simulink model "Model_6DOF_B3_2019a"  (R2019a)
settings: Solver=FixedStepAuto  StartTime=0.0  StopTime=200  FixedStep=0.05  RelTol=1e-3
values from neighbouring files (symbols this model uses):
  Ba_0 = [0 0 0 0 0 0]    [ctrl_mode_param.m]
  Bb = 4418825.3321    [load_data.m]
  Bv_0 = [tgt_speed 0 0 0 0 0]    [ctrl_mode_param.m]
  Bx_0 = [0 0 tgt_depth 0 0 0]    [ctrl_mode_param.m]
  check_angle = 10    [ctrl_mode_param.m]
  dX_imposed = 10    [ctrl_mode_param.m]
  Ixx = 5.23e7    (= 52300000)    [load_data.m]
  Ixy = 0    [load_data.m]
  Ixz = 0    [load_data.m]
  Iyy = 1.375e9    (= 1375000000)    [load_data.m]
  Iyz = 0    [load_data.m]
  Izz = 1.367e9    (= 1367000000)    [load_data.m]
  Mb = 4418825.3321    [load_data.m]
  Seastate = 5    [ctrl_mode_param.m]    (also in run.m = 0)
  Xb = 0    [load_data.m]
  Xg = 0    [load_data.m]
  Yb = 0    [load_data.m]
  Yg = 0    [load_data.m]
  Zb = 0.4406    [load_data.m]
  Zg = 0    [load_data.m]
undefined symbols (not defined in the file or in its folder): dA_BP1, dA_BP2, dA_Hull, dA_PH, dA_Sail, dA_SProot, dA_X1a, dA_X1b, dA_X2a, dA_X2b, dA_X3a, dA_X3b, dA_X4a, dA_X4b, DoF_switch, fwrite, its, LCG_switch, m_switch, mass_switch, n_BP1, n_BP2, n_Hull, n_imposed, n_PH, n_Sail, n_SProot, n_switch, n_X1a, n_X1b, n_X2a, n_X2b, n_X3a, n_X3b, n_X4a, n_X4b, nt_BP1, nt_BP2, nt_Hull, nt_PH, nt_Sail, nt_SProot, nt_X1a, nt_X1b, nt_X2a, nt_X2b, nt_X3a, nt_X3b, nt_X4a, nt_X4b, sail_switch, target_pitch, target_y, target_yaw, target_z, Usp, vt1_BP1, vt1_BP2, vt1_Hull, vt1_PH ... (+38)
libraries: simulink x5
(part 2 of 6)

== system Model_6DOF_B3_2019a/HDM/HDM B3/Wave, Virtual Mass and Hydrostatic ==
  Bx_earth : Inport
  Bv_ship : Inport  Port=2
  SeaState : Inport  Port=3
  dLCG : Inport  Port=4
  Ba_ship : Inport  Port=5
  dX_CTRL : Inport  Port=6
  fwrite : Inport  Port=7
  Add : Sum  Inputs=+-
  CG : Constant  Value=[32.3114 0 0]
  CGi : Constant  Value=|
      | [5.0784E+00	0.0000E+00	8.0728E-03;
      | 1.1013E+01	0.0000E+00	2.5384E-01;
      | 1.7302E+01	0.0000E+00	3.0728E-01;
      | 2.5741E+01	0.0000E+00	4.1417E-01;
      | 3.4688E+01	0.0000E+00	4.1585E-01;
      | 4.2324E+01	0.0000E+00	3.2444E-01;
      | 4.9992E+01	0.0000E+00	3.3454E-01;
      | 5.7427E+01	0.0000E+00	1.7420E-02;
      | 6.3078E+01	0.0000E+00	1.8824E-02;
      | 6.6703E+01	0.0000E+00	1.1340E-02;
      | 2.5141E+01	0.0000E+00	8.6491E+00;
      | 2.1732E+01	0.0000E+00	9.7273E+00;
      | 6.3166E+01	0.0000E+00	-4.0823E-17;
      | 2.2043E+01	0.0000E+00	9.7261E+00;
      | 6.3451E+01	0.0000E+00	-6.2238E-17;
      | ]
  Cvm*dm : Constant  Value=|
      | [8.4658E+04	1.7229E+05	1.6487E+05
      | 2.3551E+04	4.3394E+05	3.6176E+05
      | 1.1585E+03	5.9767E+05	4.2996E+05
      | 1.4123E+02	1.1354E+06	6.5606E+05
      | 9.1503E+01	6.9712E+05	5.1688E+05
      | 9.6110E+01	6.7201E+05	5.1905E+05
      | 1.2163E+04	5.7818E+05	4.7547E+05
      | 3.7219E+04	3.4697E+05	3.3508E+05
      | 1.9318E+04	7.7284E+04	7.6560E+04
      | 1.5368E+04	2.6375E+04	2.6268E+04
      | 1.8312E+04	4.5870E+05	5.1108E+04
      | 3.1859E+02	1.2645E+04	3.4886E+02
      | 3.0285E+03	4.4945E+04	4.4489E+04
      | 7.9160E+02	8.8963E+02	1.3306E+04
      | 1.2115E+03	3.9547E+04	3.9205E+04
      | ]
  Demux : Demux  Outputs=3
  Demux1 : Demux  Outputs=3
  Derivative : Derivative
  Derivative1 : Derivative
  Gain : Gain
  MATLAB Function : MATLAB Function  TreatAsAtomicUnit=on
  MATLAB Function1 : MATLAB Function  TreatAsAtomicUnit=on
  Manual Switch : ManualSwitch
  Wave Particle Motions : Subsystem
  Xvm : Outport
  Yvm : Outport  Port=2
  Zvm : Outport  Port=3
  Kvm : Outport  Port=4
  Mvm : Outport  Port=5
  Nvm : Outport  Port=6
  z_eff : Outport  Port=7
  uwsXi : Outport  Port=8
  uwsCG : Outport  Port=9
  B_FM : Outport  Port=10
  wires:
  Wave Particle Motions/2(zeff) -> z_eff/1
  Bx_earth/1 -> Wave Particle Motions/2(X_earth)
  CGi/1 -> Wave Particle Motions/3(CGi)
  CG/1 -> Wave Particle Motions/4(CG)
  Wave Particle Motions/1(Rs) -> MATLAB Function/3(Rs)
  SeaState/1 -> Wave Particle Motions/5(SeaState)
  dLCG/1 -> Wave Particle Motions/6(dLCG)
  Bv_ship/1 -> Wave Particle Motions/1(U_ship)
  MATLAB Function/7(Fvm) -> Manual Switch/1  "Fvm"
  MATLAB Function/8(Mvm) -> Demux1/1  "Mvm"
  Demux/1 -> Xvm/1
  Demux/2 -> Yvm/1
  Demux/3 -> Zvm/1
  Demux1/2 -> Mvm/1
  Demux1/1 -> Kvm/1
  Demux1/3 -> Nvm/1
  Wave Particle Motions/3(uwXis) -> uwsXi/1
  Wave Particle Motions/4(uwsCG) -> uwsCG/1, Derivative/1
  Cvm*dm/1 -> Gain/1
  Derivative/1 -> MATLAB Function1/1(awsCG)
  Ba_ship/1 -> MATLAB Function1/2(asCG)
  Manual Switch/1 -> Demux/1
  MATLAB Function1/1(Fvm) -> Manual Switch/2
  Wave Particle Motions/5(uws) -> Add/1
  Wave Particle Motions/6(urs) -> Add/2
  Add/1 -> Derivative1/1
  Derivative1/1 -> MATLAB Function/2(Awrs)  "d/dt(aw-ar)"
  Wave Particle Motions/7(B_FM) -> B_FM/1
  Gain/1 -> MATLAB Function/1(cvm)
  dX_CTRL/1 -> Wave Particle Motions/7(dX_CTRL)
  fwrite/1 -> Wave Particle Motions/8(fwrite)

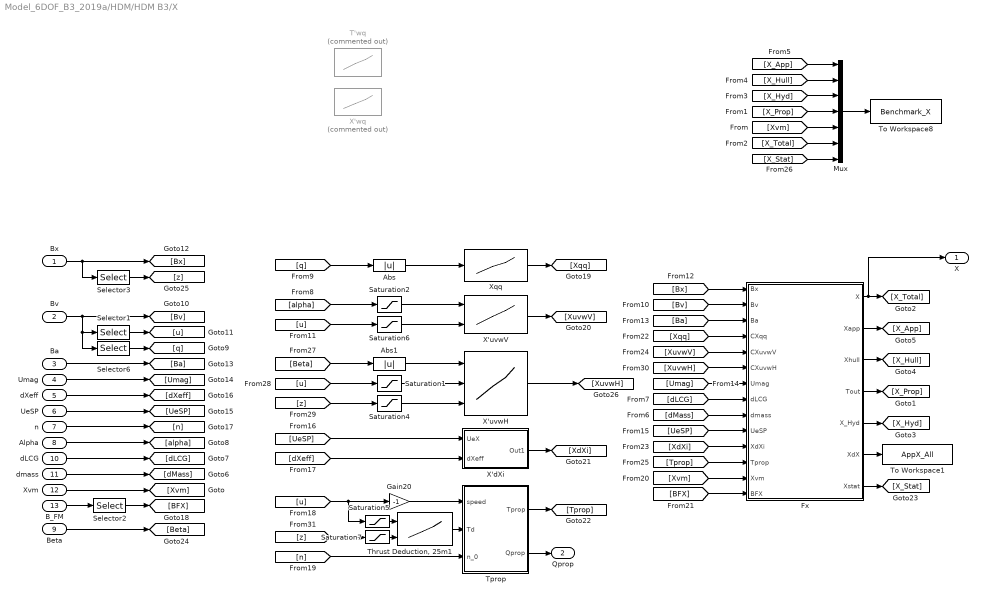
== system Model_6DOF_B3_2019a/HDM/HDM B3/X ==
  Bx : Inport
  Bv : Inport  Port=2
  Ba : Inport  Port=3
  Umag : Inport  Port=4
  dXeff : Inport  Port=5
  UeSP : Inport  Port=6
  n : Inport  Port=7
  Alpha : Inport  Port=8
  Beta : Inport  Port=9
  dLCG : Inport  Port=10
  dmass : Inport  Port=11
  Xvm : Inport  Port=12
  B_FM : Inport  Port=13
  Abs : Abs
  Abs1 : Abs
  Fx : MATLAB Function  TreatAsAtomicUnit=on
  Gain20 : Gain  Gain=-1
  Mux : Mux  Inputs=7
  Saturation1 : Saturate  UpperLimit=-1.543332  LowerLimit=-5.14444
  Saturation2 : Saturate  UpperLimit=30  LowerLimit=-30
  Saturation4 : Saturate  UpperLimit=-13.8724  LowerLimit=-35.0624
  Saturation5 : Saturate  UpperLimit=-13.8724  LowerLimit=-36.3724
  Saturation6 : Saturate  UpperLimit=-1.543332  LowerLimit=-5.14444
  Saturation7 : Saturate  UpperLimit=-1.54333333  LowerLimit=-5.14444
  Selector1 : Selector  InputPortWidth=6  IndexOptions=Index vector (dialog)  Indices=1  OutputSizes=1
  Selector2 : Selector  InputPortWidth=6  IndexOptions=Index vector (dialog)  Indices=1  OutputSizes=1
  Selector3 : Selector  InputPortWidth=6  IndexOptions=Index vector (dialog)  Indices=3  OutputSizes=1
  Selector6 : Selector  InputPortWidth=6  IndexOptions=Index vector (dialog)  Indices=5  OutputSizes=1
  T'wq : Lookup_n-D  Commented=on  BreakpointsForDimension1=|  BreakpointsForDimension2=|  Table=|  InternalRulePriority=Speed  RndMeth=Simplest  InputSameDT=on
      BreakpointsForDimension1=|
      | [-2.5000E-02
      | -2.0000E-02
      | -1.5000E-02
      | -1.0000E-02
      | -5.0000E-03
      | 0.0000E+00
      | 5.0000E-03
      | ]
      BreakpointsForDimension2=|
      | [-7.71666
      | -5.14444
      | -3.086664]
      Table=|
      | reshape([-2.7354E-04
      | -2.2597E-04
      | -1.7840E-04
      | -1.3083E-04
      | -8.3252E-05
      | -3.5680E-05
      | 1.1893E-05
      | -9.4081E-05
      | -7.5784E-05
      | -5.7487E-05
      | -3.9189E-05
      | -2.0892E-05
      | -2.5949E-06
      | 1.5702E-05
      | -1.4962E-04
      | -1.2035E-04
      | -9.1070E-05
      | -6.1795E-05
      | -3.2519E-05
      | -3.2436E-06
      | 2.6032E-05
      | ],[7,3])
  "Thrust Deduction, 25m1" : Lookup_n-D  BreakpointsForDimension1=|  BreakpointsForDimension2=[-5.14444 -3.086664 -1.543332]  Table=|  InternalRulePriority=Speed  RndMeth=Simplest  InputSameDT=on
      BreakpointsForDimension1=|
      | [-36.3724
      | -18.3724
      | -15.3724
      | -13.8724]
      Table=|
      | reshape([0.245958
      | 0.251311246
      | 0.25251
      | 0.251322
      | 0.2444134
      | 0.2498597
      | 0.2509219
      | 0.2498992
      | 0.2496
      | 0.2594532
      | 0.257802
      | 0.2475762],[4,3])
  To Workspace1 : ToWorkspace  VariableName=AppX_All  SaveFormat=Timeseries  SampleTime=-1
  To Workspace8 : ToWorkspace  VariableName=Benchmark_X  SaveFormat=Timeseries  SampleTime=-1
  Tprop : MATLAB Function  TreatAsAtomicUnit=on
  X'dXi : Subsystem
  X'uvwH : Lookup_n-D  NumberOfTableDimensions=3  BreakpointsForDimension1=|  BreakpointsForDimension2=|  BreakpointsForDimension3=|  Table=|  InternalRulePriority=Speed  RndMeth=Simplest  InputSameDT=on
      BreakpointsForDimension1=|
      | [0
      | 4
      | 8
      | 12]
      BreakpointsForDimension2=|
      | [-5.1444
      | -3.08664
      | -1.54332]
      Table=|
      | reshape([0.0000000E+00
      | 8.7490400E-05
      | -4.2970032E-04
      | -8.6882993E-04
      | 0.0000000E+00
      | 9.2255510E-05
      | -3.6462757E-04
      | -8.6516720E-04
      | 0.0000000E+00
      | -8.0508235E-05
      | -3.3610820E-04
      | -9.1603355E-04
      | 0.0000000E+00
      | -9.0915847E-05
      | -3.9252667E-04
      | -9.2068441E-04
      | 0.0000000E+00
      | -1.0407599E-04
      | -3.8836462E-04
      | -9.1865822E-04
      | 0.0000000E+00
      | -8.4723950E-05
      | -3.5324770E-04
      | -9.7126434E-04
      | 0.0000000E+00
      | -9.3766627E-05
      | -4.1342843E-04
      | -9.4161914E-04
      | 0.0000000E+00
      | -1.0916277E-04
      | -4.0683220E-04
      | -9.6707684E-04
      | 0.0000000E+00
      | -8.8664811E-05
      | -3.7605406E-04
      | -9.4194453E-04
      | 0.0000000E+00
      | -9.2876985E-05
      | -4.0365964E-04
      | -9.3239814E-04
      | 0.0000000E+00
      | -1.1414747E-04
      | -4.4323139E-04
      | -1.0049645E-03
      | 0.0000000E+00
      | -9.4615234E-05
      | -4.9251136E-04
      | -9.8471513E-04],[4,3,4])
      BreakpointsForDimension3=|
      | [-35.0624 -18.3724 -15.3724 -13.8724
      | ]
  X'uvwV : Lookup_n-D  BreakpointsForDimension1=|  BreakpointsForDimension2=|  Table=|  InternalRulePriority=Speed  RndMeth=Simplest  InputSameDT=on
      BreakpointsForDimension1=|
      | [-12
      | -8
      | -4
      | 0
      | 4
      | 8
      | 12]
      BreakpointsForDimension2=|
      | [-5.1444
      | -3.08664
      | -1.54332]
      Table=|
      | reshape([8.5556500E-04
      | 9.0045500E-04
      | 9.7379500E-04
      | 1.0292250E-03
      | 1.0286950E-03
      | 9.7963500E-04
      | 1.0147450E-03
      | 9.0637500E-04
      | 9.3710500E-04
      | 1.0133950E-03
      | 1.0723650E-03
      | 1.0693650E-03
      | 1.0284650E-03
      | 1.1084650E-03
      | 9.8653120E-04
      | 9.9350120E-04
      | 1.0534412E-03
      | 1.1098412E-03
      | 1.1115412E-03
      | 1.0836412E-03
      | 1.1582412E-03],[7,3])
  X'wq : Lookup_n-D  Commented=on  BreakpointsForDimension1=|  BreakpointsForDimension2=[-7.71666 -5.14444 -3.086664 -1.543332]  Table=|  InternalRulePriority=Speed  RndMeth=Simplest  InputSameDT=on
      BreakpointsForDimension1=|
      | [-2.5000E-02
      | -2.0000E-02
      | -1.5000E-02
      | -1.0000E-02
      | -5.0000E-03
      | 0.0000E+00
      | 5.0000E-03
      | ]
      Table=|
      | reshape([2.0716E-04
      | 1.9060E-04
      | 1.7404E-04
      | 1.5748E-04
      | 1.4091E-04
      | 1.2435E-04
      | 1.0779E-04
      | 1.3610E-04
      | 1.1954E-04
      | 1.0298E-04
      | 8.6416E-05
      | 6.9855E-05
      | 5.3295E-05
      | 3.6734E-05
      | 1.5577E-04
      | 1.2817E-04
      | 1.0057E-04
      | 7.2967E-05
      | 4.5366E-05
      | 1.7765E-05
      | -9.8361E-06
      | 1.4245E-04
      | 1.1485E-04
      | 8.7244E-05
      | 5.9643E-05
      | 3.2042E-05
      | 4.4412E-06
      | -2.3160E-05
      | ],[7,4])
  Xqq : Lookup_n-D  NumberOfTableDimensions=1  BreakpointsForDimension1=|  Table=|  InternalRulePriority=Speed  RndMeth=Simplest  InputSameDT=on
      BreakpointsForDimension1=|
      | [-0.02
      | -0.015
      | -0.012958963
      | -0.009719222
      | -0.006479482
      | -0.003239741
      | -0.00161987
      | -0.000647948
      | 0.000647948
      | 0.00161987
      | 0.003239741
      | 0.006479482
      | 0.009719222
      | 0.012958963
      | 0.015
      | 0.02
      | ]
      Table=|
      | [1.5581E-04
      | 1.1369E-04
      | 2.0348E-04
      | 4.5268E-04
      | 3.8456E-04
      | 9.9241E-05
      | 3.8998E-04
      | 9.1300E-05
      | -3.1574E-04
      | -7.9139E-05
      | -9.0517E-04
      | -4.4764E-04
      | -5.9612E-04
      | -5.5873E-04
      | -5.9343E-04
      | -5.5869E-04
      | ]
  X : Outport
  Qprop : Outport  Port=2
  wires:
  Saturation2/1 -> X'uvwV/1
  Gain20/1 -> Tprop/1(speed)
  Fx/1(X) -> [X_Total], X/1
  [u] -> Saturation5/1, Gain20/1
  [q] -> Abs/1
  Abs/1 -> Xqq/1
  "Thrust Deduction, 25m1"/1 -> Tprop/2(Td)
  Saturation6/1 -> X'uvwV/2
  Mux/1 -> To Workspace8/1
  Fx/6(XdX) -> To Workspace1/1
  B_FM/1 -> Selector2/1
  Fx/7(Xstat) -> [X_Stat]
  [Xvm] -> Mux/5
  Fx/4(Tout) -> [X_Prop]
  [X_Prop] -> Mux/4
  [X_Total] -> Mux/6
  [X_Hyd] -> Mux/3
  Fx/5(X_Hyd) -> [X_Hyd]
  [X_Hull] -> Mux/2
  Fx/3(Xhull) -> [X_Hull]
  Fx/2(Xapp) -> [X_App]
  [X_App] -> Mux/1
  [dMass] -> Fx/9(dmass)
  dmass/1 -> [dMass]
  [dLCG] -> Fx/8(dLCG)
  dLCG/1 -> [dLCG]
  [alpha] -> Saturation2/1
  Alpha/1 -> [alpha]
  Bv/1 -> [Bv], Selector6/1, Selector1/1
  Selector6/1 -> [q]
  [Bv] -> Fx/2(Bv)
  [u] -> Saturation6/1
  Selector1/1 -> [u]
  [Bx] -> Fx/1(Bx)
  Bx/1 -> [Bx], Selector3/1
  [Ba] -> Fx/3(Ba)
  Ba/1 -> [Ba]
  [Umag] -> Fx/7(Umag)
  Umag/1 -> [Umag]
  [UeSP] -> Fx/10(UeSP)
  UeSP/1 -> [UeSP]
  [UeSP] -> X'dXi/1(UeX)
  [dXeff] -> X'dXi/2(dXeff)
  dXeff/1 -> [dXeff]
  n/1 -> [n]
  [n] -> Tprop/3(n_0)
  Xvm/1 -> [Xvm]
  [Xvm] -> Fx/13(Xvm)
  Selector2/1 -> [BFX]
  [BFX] -> Fx/14(BFX)
  [Xqq] -> Fx/4(CXqq)
  Xqq/1 -> [Xqq]
  X'uvwV/1 -> [XuvwV]
  X'dXi/1(Out1) -> [XdXi]
  [XdXi] -> Fx/11(XdXi)
  [XuvwV] -> Fx/5(CXuvwV)
  Tprop/1(Tprop) -> [Tprop]
  [Tprop] -> Fx/12(Tprop)
  [X_Stat] -> Mux/7
  Beta/1 -> [Beta]
  Abs1/1 -> X'uvwH/1
  [Beta] -> Abs1/1
  [u] -> Saturation1/1
  Saturation1/1 -> X'uvwH/2
  Selector3/1 -> [z]
  [z] -> Saturation4/1
  Saturation4/1 -> X'uvwH/3
  X'uvwH/1 -> [XuvwH]
  [XuvwH] -> Fx/6(CXuvwH)
  Saturation5/1 -> "Thrust Deduction, 25m1"/1
  Saturation7/1 -> "Thrust Deduction, 25m1"/2
  [z] -> Saturation7/1
  Tprop/2(Qprop) -> Qprop/1

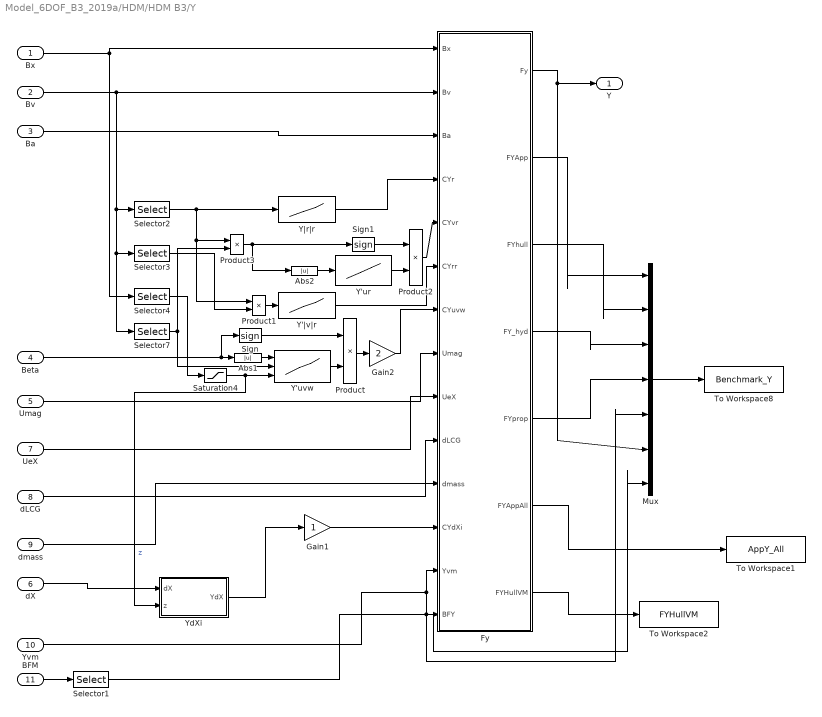
== system Model_6DOF_B3_2019a/HDM/HDM B3/Y ==
  Bx : Inport
  Bv : Inport  Port=2
  Ba : Inport  Port=3
  Beta : Inport  Port=4
  Umag : Inport  Port=5
  dX : Inport  Port=6
  UeX : Inport  Port=7
  dLCG : Inport  Port=8
  dmass : Inport  Port=9
  Yvm : Inport  Port=10
  BFM : Inport  Port=11
  Abs1 : Abs
  Abs2 : Abs
  Fy : MATLAB Function  TreatAsAtomicUnit=on
  Gain1 : Gain
  Gain2 : Gain  Gain=2
  Mux : Mux  Inputs=7
  Product{,1..3} (4 alike) : Product
  Saturation4 : Saturate  UpperLimit=-13.8724  LowerLimit=-35.0624
  Selector1 : Selector  InputPortWidth=6  IndexOptions=Index vector (dialog)  Indices=2  OutputSizes=1
  Selector2 : Selector  InputPortWidth=6  IndexOptions=Index vector (dialog)  Indices=6  OutputSizes=1
  Selector3 : Selector  InputPortWidth=6  IndexOptions=Index vector (dialog)  Indices=2  OutputSizes=1
  Selector4 : Selector  InputPortWidth=6  IndexOptions=Index vector (dialog)  Indices=3  OutputSizes=1
  Selector7 : Selector  InputPortWidth=6  IndexOptions=Index vector (dialog)  Indices=1  OutputSizes=1
  Sign : Signum
  Sign1 : Signum
  To Workspace1 : ToWorkspace  VariableName=AppY_All  SaveFormat=Timeseries  SampleTime=-1
  To Workspace2 : ToWorkspace  VariableName=FYHullVM  SaveFormat=Timeseries  SampleTime=-1
  To Workspace8 : ToWorkspace  VariableName=Benchmark_Y  SaveFormat=Timeseries  SampleTime=-1
  Y'ur : Lookup_n-D  NumberOfTableDimensions=1  BreakpointsForDimension1=|  Table=|  InternalRulePriority=Speed  RndMeth=Simplest  InputSameDT=on
      BreakpointsForDimension1=|
      | [0.03999989
      | 0.079999993
      | 0.11999963
      | 0.15999956]
      Table=|
      | [-5.2094E-04
      | -1.0594E-03
      | -1.5649E-03
      | -2.0981E-03]
  Y'uvw : Lookup_n-D  NumberOfTableDimensions=3  BreakpointsForDimension1=|  BreakpointsForDimension2=|  BreakpointsForDimension3=|  Table=|  InternalRulePriority=Speed  RndMeth=Simplest  InputSameDT=on
      BreakpointsForDimension1=|
      | [0
      | 4
      | 8
      | 12]
      BreakpointsForDimension2=|
      | [-5.1444E+00
      | -3.0866E+00
      | -1.5433E+00
      | ]
      Table=|
      | reshape([0.0000000E+00
      | -5.0280621E-03
      | -9.4175348E-03
      | -1.4397458E-02
      | 0.0000000E+00
      | -5.0037454E-03
      | -9.1645405E-03
      | -1.4507402E-02
      | 0.0000000E+00
      | -4.2819107E-03
      | -9.0361786E-03
      | -1.4507235E-02
      | 0.0000000E+00
      | -4.7723270E-03
      | -9.7378407E-03
      | -1.5377541E-02
      | 0.0000000E+00
      | -4.7276301E-03
      | -9.6949815E-03
      | -1.5393721E-02
      | 0.0000000E+00
      | -4.5359209E-03
      | -9.4966039E-03
      | -1.6947859E-02
      | 0.0000000E+00
      | -5.1295007E-03
      | -1.0575377E-02
      | -1.6672924E-02
      | 0.0000000E+00
      | -4.9811404E-03
      | -1.0209461E-02
      | -1.6298327E-02
      | 0.0000000E+00
      | -4.7780219E-03
      | -1.0008968E-02
      | -1.6115181E-02
      | 0.0000000E+00
      | -5.7252015E-03
      | -1.1973447E-02
      | -1.9152812E-02
      | 0.0000000E+00
      | -5.2128737E-03
      | -1.0845978E-02
      | -1.7281669E-02
      | 0.0000000E+00
      | -4.9979037E-03
      | -1.0845685E-02
      | -1.6944141E-02],[4,3,4])
      BreakpointsForDimension3=|
      | [-35.0624 -18.3724 -15.3724 -13.8724
      | ]
  Y'|v|r : Lookup_n-D  NumberOfTableDimensions=1  BreakpointsForDimension1=|  Table=|  InternalRulePriority=Speed  RndMeth=Simplest  InputSameDT=on
      BreakpointsForDimension1=|
      | [-0.0015
      | -0.0012
      | -0.0009
      | -0.0006
      | -0.0003
      | -0.0001
      | 0.0001
      | 0.0003
      | 0.0006
      | 0.0009
      | 0.0012
      | 0.0015]
      Table=|
      | [-2.9784E-01
      | -2.6725E-01
      | -2.3292E-01
      | -2.0077E-01
      | -1.1489E-01
      | -7.6673E-03
      | -7.5516E-03
      | -1.1617E-01
      | -2.0077E-01
      | -2.9128E-01
      | -3.5974E-01
      | -4.7839E-01]
  YdXi : Subsystem
  Y|r|r : Lookup_n-D  NumberOfTableDimensions=1  BreakpointsForDimension1=|  Table=|  InternalRulePriority=Speed  RndMeth=Simplest  InputSameDT=on
      BreakpointsForDimension1=|
      | [-0.02
      | -0.015
      | -0.012958963
      | -0.009719222
      | -0.006479482
      | -0.003239741
      | -0.00161987
      | -0.000647948
      | 0.000647948
      | 0.00161987
      | 0.003239741
      | 0.006479482
      | 0.009719222
      | 0.012958963
      | 0.015
      | 0.02
      | ]
      Table=|
      | [3.6478E-03
      | 3.8686E-03
      | 3.4313E-03
      | 4.0790E-03
      | 3.9500E-03
      | 3.6018E-03
      | 3.6796E-03
      | 3.5502E-03
      | 3.4310E-03
      | 3.4872E-03
      | 4.2239E-03
      | 4.0934E-03
      | 3.0314E-03
      | 2.5726E-03
      | 2.9188E-03
      | 2.7740E-03
      | ]
  Y : Outport
  wires:
  Selector7/1 -> Product3/2, Y'uvw/2
  Beta/1 -> Sign/1, Abs1/1
  Bv/1 -> Selector7/1, Selector3/1, Selector2/1, Fy/2(Bv)
  Umag/1 -> Fy/8(Umag)
  Bx/1 -> Selector4/1, Fy/1(Bx)
  UeX/1 -> Fy/9(UeX)
  Selector3/1 -> Product1/2
  Ba/1 -> Fy/3(Ba)
  dLCG/1 -> Fy/10(dLCG)
  dmass/1 -> Fy/11(dmass)
  dX/1 -> YdXi/1(dX)
  Product3/1 -> Abs2/1, Sign1/1
  Product1/1 -> Y'|v|r/1
  Selector2/1 -> Product1/1, Product3/1, Y|r|r/1
  Y'|v|r/1 -> Fy/6(CYrr)
  Fy/1(Fy) -> Mux/6, Y/1
  Y|r|r/1 -> Fy/4(CYr)
  Y'ur/1 -> Product2/2
  Selector4/1 -> Saturation4/1
  Y'uvw/1 -> Product/2
  Sign/1 -> Product/1
  Abs1/1 -> Y'uvw/1
  Product2/1 -> Fy/5(CYvr)
  Sign1/1 -> Product2/1
  Abs2/1 -> Y'ur/1
  YdXi/1(YdX) -> Gain1/1
  Product/1 -> Gain2/1
  Gain2/1 -> Fy/7(CYuvw)
  Yvm/1 -> Mux/5, Fy/13(Yvm)
  Mux/1 -> To Workspace8/1
  Fy/2(FYApp) -> Mux/1
  Fy/3(FYhull) -> Mux/2
  Fy/4(FY_hyd) -> Mux/3
  Fy/5(FYprop) -> Mux/4
  Fy/6(FYAppAll) -> To Workspace1/1
  BFM/1 -> Selector1/1
  Selector1/1 -> Mux/7, Fy/14(BFY)
  Fy/7(FYHullVM) -> To Workspace2/1
  Saturation4/1 -> Y'uvw/3, YdXi/2(z)  "z"
  Gain1/1 -> Fy/12(CYdXi)

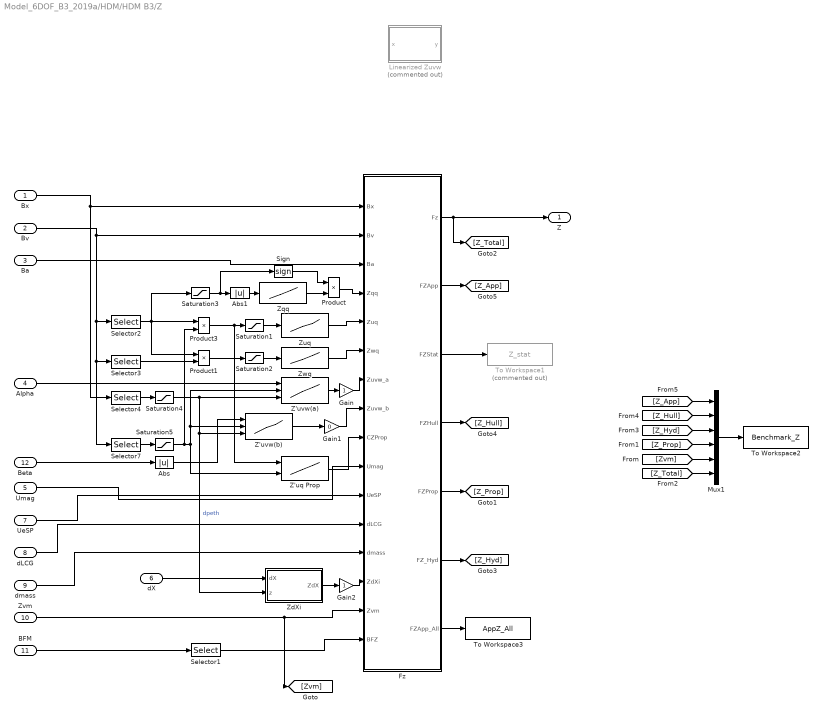
== system Model_6DOF_B3_2019a/HDM/HDM B3/Z ==
  Bx : Inport
  Bv : Inport  Port=2
  Ba : Inport  Port=3
  Alpha : Inport  Port=4
  Umag : Inport  Port=5
  dX : Inport  Port=6
  UeSP : Inport  Port=7
  dLCG : Inport  Port=8
  dmass : Inport  Port=9
  Zvm : Inport  Port=10
  BFM : Inport  Port=11
  Beta : Inport  Port=12
  Abs : Abs
  Abs1 : Abs
  Fz : MATLAB Function  TreatAsAtomicUnit=on
  Gain : Gain
  Gain1 : Gain  Gain=0
  Gain2 : Gain
  Linearized Zuvw : MATLAB Function  Commented=on  TreatAsAtomicUnit=on
  Mux1 : Mux  Inputs=6
  Product : Product
  Product1 : Product
  Product3 : Product
  Saturation1 : Saturate  UpperLimit=0.04  LowerLimit=-0.04
  Saturation2 : Saturate  UpperLimit=0.0015  LowerLimit=-0.0015
  Saturation3 : Saturate  UpperLimit=0.02  LowerLimit=-0.02
  Saturation4 : Saturate  UpperLimit=-13.8724  LowerLimit=-35.0624
  Saturation5 : Saturate  UpperLimit=-1.5433E+00  LowerLimit=-5.14444
  Selector1 : Selector  InputPortWidth=6  IndexOptions=Index vector (dialog)  Indices=3  OutputSizes=1
  Selector2 : Selector  InputPortWidth=6  IndexOptions=Index vector (dialog)  Indices=5  OutputSizes=1
  Selector3 : Selector  InputPortWidth=6  IndexOptions=Index vector (dialog)  Indices=3  OutputSizes=1
  Selector4 : Selector  InputPortWidth=6  IndexOptions=Index vector (dialog)  Indices=3  OutputSizes=1
  Selector7 : Selector  InputPortWidth=6  IndexOptions=Index vector (dialog)  Indices=1  OutputSizes=1
  Sign : Signum
  To Workspace1 : ToWorkspace  Commented=on  VariableName=Z_stat  SaveFormat=Timeseries  SampleTime=-1
  To Workspace2 : ToWorkspace  VariableName=Benchmark_Z  SaveFormat=Timeseries  SampleTime=-1
  To Workspace3 : ToWorkspace  VariableName=AppZ_All  SaveFormat=Timeseries  SampleTime=-1
  Z'uq Prop : Lookup_n-D  BreakpointsForDimension1=|  BreakpointsForDimension2=[-7.71666 -5.14444 -3.086664 -1.543332]  Table=|  InternalRulePriority=Speed  RndMeth=Simplest  InputSameDT=on
      BreakpointsForDimension1=|
      | [-2.0E-01
      | -1.5E-01
      | -1.0E-01
      | -5.0E-02
      | 0.0E+00
      | 5.0E-02
      | 1.0E-01
      | 1.5E-01
      | 2.0E-01
      | ]
      Table=|
      | reshape([1.3913E-04
      | 1.0452E-04
      | 6.9900E-05
      | 3.5283E-05
      | 6.6700E-07
      | -3.3949E-05
      | -6.8566E-05
      | -1.0318E-04
      | -1.3780E-04
      | 2.8914E-04
      | 2.1702E-04
      | 1.4490E-04
      | 7.2785E-05
      | 6.6700E-07
      | -7.1451E-05
      | -1.4357E-04
      | -2.1569E-04
      | -2.8780E-04
      | 1.1606E-04
      | 8.7208E-05
      | 5.8361E-05
      | 2.9514E-05
      | 6.6700E-07
      | -2.8180E-05
      | -5.7027E-05
      | -8.5874E-05
      | -1.1472E-04
      | 1.1606E-04
      | 8.7208E-05
      | 5.8361E-05
      | 2.9514E-05
      | 6.6700E-07
      | -2.8180E-05
      | -5.7027E-05
      | -8.5874E-05
      | -1.1472E-04],[9,4])
  Z'uvw(a) : Lookup_n-D  NumberOfTableDimensions=3  BreakpointsForDimension1=|  BreakpointsForDimension2=|  BreakpointsForDimension3=|  Table=|  InternalRulePriority=Speed  RndMeth=Simplest  InputSameDT=on
      BreakpointsForDimension1=|
      | [-12
      | -8
      | -4
      | 0
      | 4
      | 8
      | 12]
      BreakpointsForDimension2=|
      | [-5.1444E+00
      | -3.0866E+00
      | -1.5433E+00
      | ]
      Table=|
      | reshape([-3.82587E-03
      | -2.42543E-03
      | -1.05453E-03
      | 1.94202E-04
      | 1.48991E-03
      | 3.04047E-03
      | 4.14104E-03
      | -3.76348E-03
      | -2.38508E-03
      | -9.82619E-04
      | 1.94202E-04
      | 1.47560E-03
      | 3.02863E-03
      | 4.06663E-03
      | -3.75964E-03
      | -2.29001E-03
      | -8.34074E-04
      | 1.94202E-04
      | 1.38956E-03
      | 2.91153E-03
      | 4.15251E-03
      | -3.11218E-03
      | -1.80502E-03
      | -4.97855E-04
      | 8.09305E-04
      | 2.11647E-03
      | 3.42363E-03
      | 4.73079E-03
      | -2.62573E-03
      | -1.48072E-03
      | -3.35708E-04
      | 8.09305E-04
      | 1.95432E-03
      | 3.09933E-03
      | 4.24434E-03
      | -2.06413E-03
      | -1.10632E-03
      | -1.48507E-04
      | 8.09305E-04
      | 1.76712E-03
      | 2.72493E-03
      | 3.68274E-03
      | -3.09997E-03
      | -1.76300E-03
      | -4.26025E-04
      | 9.10947E-04
      | 2.24792E-03
      | 3.58489E-03
      | 4.92186E-03
      | -2.49055E-03
      | -1.35672E-03
      | -2.22886E-04
      | 9.10947E-04
      | 2.04478E-03
      | 3.17861E-03
      | 4.31245E-03
      | -2.64104E-03
      | -1.45704E-03
      | -2.73048E-04
      | 9.10947E-04
      | 2.09494E-03
      | 3.27894E-03
      | 4.46293E-03
      | -0.003059752
      | -0.001711935
      | -0.000364117
      | 0.0009837
      | 0.002331518
      | 0.003679335
      | 0.005027153
      | -0.002351082
      | -0.0012256
      | -0.000100118
      | 0.0009837
      | 0.002109182
      | 0.003234664
      | 0.004360146
      | -0.001725739
      | -0.000822593
      | 8.05539E-05
      | 0.0009837
      | 0.001886847
      | 0.002789993
      | 0.00369314],[7,3,4])
      BreakpointsForDimension3=|
      | [-35.0624 -18.3724 -15.3724 -13.8724
      | ]
  Z'uvw(b) : Lookup_n-D  NumberOfTableDimensions=3  BreakpointsForDimension1=|  BreakpointsForDimension2=|  BreakpointsForDimension3=|  Table=|  InternalRulePriority=Speed  RndMeth=Simplest  InputSameDT=on
      BreakpointsForDimension1=|
      | [0
      | 4
      | 8
      | 12]
      BreakpointsForDimension2=|
      | [-5.1444E+00
      | -3.0866E+00
      | -1.5433E+00
      | ]
      Table=|
      | reshape([0.0000000E+00
      | -5.9986916E-04
      | -2.7503348E-03
      | -5.0777589E-03
      | 0.0000000E+00
      | -6.0654884E-04
      | -2.4512564E-03
      | -5.2464901E-03
      | 0.0000000E+00
      | -7.6137528E-04
      | -2.4084463E-03
      | -5.2118678E-03
      | 0.0000000E+00
      | -8.2427914E-04
      | -2.5250249E-03
      | -5.3103563E-03
      | 0.0000000E+00
      | -8.1036019E-04
      | -2.5315266E-03
      | -5.5141459E-03
      | 0.0000000E+00
      | -7.9799041E-04
      | -2.5595242E-03
      | -5.2319004E-03
      | 0.0000000E+00
      | -8.6989011E-04
      | -2.5865820E-03
      | -5.6151595E-03
      | 0.0000000E+00
      | -8.4361582E-04
      | -2.6124115E-03
      | -5.7143353E-03
      | 0.0000000E+00
      | -8.2567611E-04
      | -2.6088331E-03
      | -5.6150660E-03
      | 0.0000000E+00
      | -9.1003224E-04
      | -2.7683191E-03
      | -6.0189061E-03
      | 0.0000000E+00
      | -8.4211433E-04
      | -2.5899187E-03
      | -5.7497784E-03
      | 0.0000000E+00
      | -8.2014014E-04
      | -2.4092466E-03
      | -5.6643347E-03],[4,3,4])
      BreakpointsForDimension3=|
      | [-35.0624 -18.3724 -15.3724 -13.8724
      | ]
  ZdXi : Subsystem
  Zqq : Lookup_n-D  NumberOfTableDimensions=1  BreakpointsForDimension1=|  Table=|  InternalRulePriority=Speed  RndMeth=Simplest  InputSameDT=on
      BreakpointsForDimension1=|
      | [0.000127901
      | 0.000383704
      | 0.000639507
      | 0.001279013
      | 0.002558026
      | ]
      Table=|
      | [-1.5611E-03
      | -1.0379E-04
      | 3.9238E-05
      | 1.1475E-04
      | 1.3579E-04
      | ]
  Zuq : Lookup_n-D  NumberOfTableDimensions=1  BreakpointsForDimension1=|  Table=|  InternalRulePriority=Speed  RndMeth=Simplest  InputSameDT=on
      BreakpointsForDimension1=|
      | [-0.04
      | -0.03
      | -0.02
      | -0.01
      | -0.005
      | -0.002
      | 0.002
      | 0.005
      | 0.01
      | 0.02
      | 0.03
      | 0.04
      | ]
      Table=|
      | [-9.8908E-03
      | -9.0784E-03
      | -8.9566E-03
      | -1.0733E-02
      | -1.4141E-02
      | -2.4189E-02
      | -6.5605E-03
      | -7.1594E-03
      | -7.6366E-03
      | -7.9008E-03
      | -6.1794E-03
      | -6.1029E-03
      | ]
  Zwq : Lookup_n-D  NumberOfTableDimensions=1  BreakpointsForDimension1=|  Table=|  InternalRulePriority=Speed  RndMeth=Simplest  InputSameDT=on
      BreakpointsForDimension1=|
      | [-0.0015
      | -0.0012
      | -0.0009
      | -0.0006
      | -0.0003
      | -0.0001
      | 0.0001
      | 0.0003
      | 0.0006
      | 0.0009
      | 0.0012
      | 0.0015]
      Table=|
      | [-2.9784E-01
      | -2.6725E-01
      | -2.3292E-01
      | -2.0077E-01
      | -1.1489E-01
      | -7.6673E-03
      | -7.5516E-03
      | -1.1617E-01
      | -2.0077E-01
      | -2.9128E-01
      | -3.5974E-01
      | -4.7839E-01]
  Z : Outport
  wires:
  Z'uvw(a)/1 -> Gain/1
  Selector4/1 -> Saturation4/1
  Zvm/1 -> Fz/15(Zvm), [Zvm]
  Ba/1 -> Fz/3(Ba)
  Zuq/1 -> Fz/5(Zuq)
  Fz/1(Fz) -> Z/1, [Z_Total]
  Saturation3/1 -> Sign/1, Abs1/1
  Saturation2/1 -> Zwq/1
  Saturation1/1 -> Zuq/1
  dX/1 -> ZdXi/1(dX)
  dmass/1 -> Fz/13(dmass)
  dLCG/1 -> Fz/12(dLCG)
  Product1/1 -> Saturation2/1
  Selector3/1 -> Product1/2
  UeSP/1 -> Fz/11(UeSP)
  Product3/1 -> Z'uq Prop/1, Saturation1/1
  Bx/1 -> Selector4/1, Fz/1(Bx)
  Umag/1 -> Fz/10(Umag)
  Bv/1 -> Selector2/1, Selector3/1, Selector7/1, Fz/2(Bv)
  Alpha/1 -> Z'uvw(a)/1
  Selector2/1 -> Product3/1, Saturation3/1, Product1/1
  Zwq/1 -> Fz/6(Zwq)
  Z'uq Prop/1 -> Fz/9(CZProp)
  Zqq/1 -> Product/2
  Gain/1 -> Fz/7(Zuvw_a)
  Fz/3(FZStat) -> To Workspace1/1
  BFM/1 -> Selector1/1
  Selector1/1 -> Fz/16(BFZ)
  Gain2/1 -> Fz/14(ZdXi)
  [Z_Hull] -> Mux1/2
  [Z_App] -> Mux1/1
  Mux1/1 -> To Workspace2/1
  [Z_Prop] -> Mux1/4
  [Z_Total] -> Mux1/6
  [Z_Hyd] -> Mux1/3
  [Zvm] -> Mux1/5
  Fz/2(FZApp) -> [Z_App]
  Fz/4(FZHull) -> [Z_Hull]
  Fz/5(FZProp) -> [Z_Prop]
  Fz/6(FZ_Hyd) -> [Z_Hyd]
  ZdXi/1(ZdX) -> Gain2/1
  Saturation4/1 -> ZdXi/2(z), Z'uvw(b)/3, Z'uvw(a)/3  "dpeth"
  Saturation5/1 -> Product3/2, Z'uvw(b)/2, Z'uvw(a)/2, Z'uq Prop/2
  Selector7/1 -> Saturation5/1
  Fz/7(FZApp_All) -> To Workspace3/1
  Beta/1 -> Abs/1
  Abs/1 -> Z'uvw(b)/1
  Z'uvw(b)/1 -> Gain1/1
  Gain1/1 -> Fz/8(Zuvw_b)
  Abs1/1 -> Zqq/1
  Sign/1 -> Product/1
  Product/1 -> Fz/4(Zqq)

== system Model_6DOF_B3_2019a/HDM/Integration and Coord. Transfrom/Coordinate Transform ==
  Bv : Inport
  Integrator : Integrator  InitialCondition=Bx_0
  MATLAB Function2 : MATLAB Function  TreatAsAtomicUnit=on
  X_earth : Outport  VectorParamsAs1DForOutWhenUnconnected=off
  wires:
  Bv/1 -> MATLAB Function2/2(Bv)
  MATLAB Function2/1(out) -> Integrator/1
  Integrator/1 -> X_earth/1, MATLAB Function2/1(Bx)

== system Model_6DOF_B3_2019a/HDM/Integration and Coord. Transfrom/Rigid Body Motion ==
  F_hyd : Inport
  Bx : Inport  Port=2
  Demux : Demux  Outputs=6
  Demux1 : Demux  Outputs=6
  Demux2 : Demux  Outputs=5
  Gain2 : Gain
  Integrator : Integrator  InitialCondition=Bv_0
  MATLAB Function2 : MATLAB Function  TreatAsAtomicUnit=on
  Memory1 : Memory  InitialCondition=Ba_0
  Mux1 : Mux  Inputs=6
  Mux2 : Mux  Inputs=5
  Bv : Outport  VectorParamsAs1DForOutWhenUnconnected=off
  Ba : Outport  Port=2  VectorParamsAs1DForOutWhenUnconnected=off
  wires:
  Bx/1 -> MATLAB Function2/7(bx)
  MATLAB Function2/1(out) -> Integrator/1, Memory1/1
  Integrator/1 -> MATLAB Function2/8(bv), Demux1/1
  Memory1/1 -> Ba/1
  Demux/1 -> MATLAB Function2/1(X)
  Demux/2 -> MATLAB Function2/2(Y)
  Demux/3 -> MATLAB Function2/3(Z)
  Demux/4 -> MATLAB Function2/4(K)
  Demux/5 -> MATLAB Function2/5(M)
  Demux/6 -> MATLAB Function2/6(N)
  F_hyd/1 -> Demux/1
  Demux2/3 -> Mux1/4
  Demux1/3 -> Mux2/2
  Mux2/1 -> Gain2/1
  Demux2/5 -> Mux1/6
  Demux2/2 -> Mux1/3
  Demux2/4 -> Mux1/5
  Demux1/1 -> Mux1/1
  Demux2/1 -> Mux1/2
  Demux1/5 -> Mux2/4
  Demux1/6 -> Mux2/5
  Demux1/4 -> Mux2/3
  Demux1/2 -> Mux2/1
  Gain2/1 -> Demux2/1
  Mux1/1 -> Bv/1

== system Model_6DOF_B3_2019a/HDM/HDM B3/K/KdXi ==
  dX : Inport
  UeX : Inport  Port=2
  z : Inport  Port=3
  KdX1 : Lookup_n-D  NumberOfTableDimensions=3  BreakpointsForDimension1=[-10 0 10]  BreakpointsForDimension2=|  BreakpointsForDimension3=[-5.14444 -3.08666664 -1.54332]  Table=|  InternalRulePriority=Speed  RndMeth=Simplest  InputSameDT=on
      BreakpointsForDimension2=|
      | [-36.4062987
      | -18.4062987
      | -15.4062987
      | -13.9062987]
      Table=|
      | reshape([-3.9047E-05
      | 4.5684E-07
      | 3.9769E-05
      | -3.8309E-05
      | 1.2643E-06
      | 4.0809E-05
      | -3.0256E-05
      | 1.2643E-06
      | 4.8387E-05
      | -3.7558E-05
      | 2.1545E-06
      | 4.2083E-05
      | -3.9057E-05
      | 3.6064E-07
      | 3.9562E-05
      | -3.8473E-05
      | 1.0476E-06
      | 4.0437E-05
      | -3.0256E-05
      | 1.4418E-06
      | 4.8387E-05
      | -3.7906E-05
      | 1.7415E-06
      | 4.1434E-05
      | -3.8945E-05
      | 2.8249E-07
      | 3.9429E-05
      | -3.8396E-05
      | 9.1134E-07
      | 4.0237E-05
      | -3.8190E-05
      | 9.1134E-07
      | 4.0733E-05
      | -3.7932E-05
      | 1.5343E-06
      | 4.1020E-05
      | ],[3,4,3])
  KdX2 : Lookup_n-D  NumberOfTableDimensions=3  BreakpointsForDimension1=[-10 0 10]  BreakpointsForDimension2=|  BreakpointsForDimension3=[-5.14444 -3.08666664 -1.54332]  Table=|  InternalRulePriority=Speed  RndMeth=Simplest  InputSameDT=on
      BreakpointsForDimension2=|
      | [-36.4062987
      | -18.4062987
      | -15.4062987
      | -13.9062987]
      Table=|
      | reshape([-3.5775E-05
      | -2.4080E-07
      | 3.3150E-05
      | -3.4263E-05
      | 1.2268E-06
      | 3.5342E-05
      | -2.3577E-05
      | 1.2268E-06
      | 4.6338E-05
      | -3.2368E-05
      | 3.5682E-06
      | 3.9469E-05
      | -3.5785E-05
      | -3.3131E-07
      | 3.3067E-05
      | -3.4544E-05
      | 8.9010E-07
      | 3.4889E-05
      | -2.3577E-05
      | 1.7076E-06
      | 4.6338E-05
      | -3.3141E-05
      | 2.4187E-06
      | 3.7389E-05
      | -3.5809E-05
      | -5.7189E-07
      | 3.3046E-05
      | -3.4706E-05
      | 4.2723E-07
      | 3.4588E-05
      | -3.4017E-05
      | 4.2723E-07
      | 3.5657E-05
      | -3.3562E-05
      | 1.6134E-06
      | 3.6605E-05
      | ],[3,4,3])
  KdX3 : Lookup_n-D  NumberOfTableDimensions=3  BreakpointsForDimension1=[-10 0 10]  BreakpointsForDimension2=|  BreakpointsForDimension3=[-5.14444 -3.08666664 -1.54332]  Table=|  InternalRulePriority=Speed  RndMeth=Simplest  InputSameDT=on
      BreakpointsForDimension2=|
      | [-36.4062987
      | -18.4062987
      | -15.4062987
      | -13.9062987]
      Table=|
      | reshape([-4.3139E-05
      | 1.7292E-07
      | 4.5001E-05
      | -4.4081E-05
      | -1.2796E-06
      | 4.2448E-05
      | -4.9749E-05
      | -1.2796E-06
      | 2.6691E-05
      | -4.5613E-05
      | -3.5861E-06
      | 3.8362E-05
      | -4.2707E-05
      | 2.7384E-07
      | 4.4575E-05
      | -4.3360E-05
      | -9.3523E-07
      | 4.2465E-05
      | -4.9749E-05
      | -1.7362E-06
      | 2.6691E-05
      | -4.4279E-05
      | -2.4363E-06
      | 3.9821E-05
      | -4.1687E-05
      | 5.3371E-07
      | 4.3082E-05
      | -4.2289E-05
      | -4.5361E-07
      | 4.1207E-05
      | -4.2616E-05
      | -4.5361E-07
      | 4.0204E-05
      | -4.2521E-05
      | -1.6159E-06
      | 3.9463E-05
      | ],[3,4,3])
  KdX4 : Lookup_n-D  NumberOfTableDimensions=3  BreakpointsForDimension1=[-10 0 10]  BreakpointsForDimension2=|  BreakpointsForDimension3=[-5.14444 -3.08666664 -1.54332]  Table=|  InternalRulePriority=Speed  RndMeth=Simplest  InputSameDT=on
      BreakpointsForDimension2=|
      | [-36.4062987
      | -18.4062987
      | -15.4062987
      | -13.9062987]
      Table=|
      | reshape([-4.0969E-05
      | -4.5313E-07
      | 4.0019E-05
      | -4.1787E-05
      | -1.2714E-06
      | 3.9006E-05
      | -4.8908E-05
      | -1.2714E-06
      | 3.0663E-05
      | -4.2681E-05
      | -2.1920E-06
      | 3.7920E-05
      | -4.0777E-05
      | -3.6185E-07
      | 4.0047E-05
      | -4.1470E-05
      | -1.0577E-06
      | 3.9147E-05
      | -4.8908E-05
      | -1.4679E-06
      | 3.0663E-05
      | -4.2187E-05
      | -1.7779E-06
      | 3.8312E-05
      | -4.0496E-05
      | -2.8854E-07
      | 4.0049E-05
      | -4.1082E-05
      | -9.2714E-07
      | 3.9223E-05
      | -4.1472E-05
      | -9.2714E-07
      | 3.8784E-05
      | -4.1733E-05
      | -1.5768E-06
      | 3.8383E-05
      | ],[3,4,3])
  Mux : Mux
  Selector1 : Selector  InputPortWidth=5  IndexOptions=Index vector (dialog)  Indices=2  OutputSizes=1
  Selector2 : Selector  InputPortWidth=5  IndexOptions=Index vector (dialog)  Indices=3  OutputSizes=1
  Selector3 : Selector  InputPortWidth=5  IndexOptions=Index vector (dialog)  Indices=4  OutputSizes=1
  Selector4 : Selector  InputPortWidth=5  IndexOptions=Index vector (dialog)  Indices=1  OutputSizes=1
  Selector5 : Selector  InputPortWidth=5  IndexOptions=Index vector (dialog)  Indices=2  OutputSizes=1
  Selector6 : Selector  InputPortWidth=5  IndexOptions=Index vector (dialog)  Indices=3  OutputSizes=1
  Selector7 : Selector  InputPortWidth=5  IndexOptions=Index vector (dialog)  Indices=1  OutputSizes=1
  Selector8 : Selector  InputPortWidth=5  IndexOptions=Index vector (dialog)  Indices=4  OutputSizes=1
  KdXi : Outport
  wires:
  dX/1 -> Selector1/1, Selector3/1, Selector2/1, Selector7/1
  Selector7/1 -> KdX1/1
  Mux/1 -> KdXi/1
  z/1 -> KdX4/2, KdX3/2, KdX2/2, KdX1/2
  KdX1/1 -> Mux/1
  KdX2/1 -> Mux/2
  KdX3/1 -> Mux/3
  KdX4/1 -> Mux/4
  Selector1/1 -> KdX2/1
  Selector2/1 -> KdX3/1
  Selector3/1 -> KdX4/1
  UeX/1 -> Selector6/1, Selector8/1, Selector5/1, Selector4/1
  Selector4/1 -> KdX1/3
  Selector8/1 -> KdX4/3
  Selector6/1 -> KdX3/3
  Selector5/1 -> KdX2/3

== system Model_6DOF_B3_2019a/HDM/HDM B3/M/Mdxi ==
  dX : Inport
  z : Inport  Port=2
  Demux6 : Demux  Outputs=5
  Gain{,1..4} (5 alike) : Gain
  Mux : Mux  Inputs=5
  ZudX1 q+1 : Lookup_n-D  BreakpointsForDimension1=[-30 -20 -10 0 10 20 30]  BreakpointsForDimension2=[-35.0624 -15.3724 -13.8724]  BreakpointsForDimension3=[-5.14444 -3.08666664 -1.54332]  Table=|  InternalRulePriority=Speed  RndMeth=Simplest  InputSameDT=on
      | reshape([0.000594819
      | 0.000394915
      | 0.000195011
      | -4.89222E-06
      | -0.000204796
      | -0.0004047
      | -0.000604603
      | 0.000596203
      | 0.000392018
      | 0.000187833
      | -1.6352E-05
      | -0.000220537
      | -0.000424722
      | -0.000628907
      | 0.000582351
      | 0.000381446
      | 0.000180542
      | -2.03625E-05
      | -0.000221267
      | -0.000422171
      | -0.000623076
      | ],[7,3])
  ZudX1 q+2 : Lookup_n-D  BreakpointsForDimension1=[-30 -20 -10 0 10 20 30]  BreakpointsForDimension2=[-35.0624 -15.3724 -13.8724]  BreakpointsForDimension3=[-5.14444 -3.08666664 -1.54332]  Table=|  InternalRulePriority=Speed  RndMeth=Simplest  InputSameDT=on
      | reshape([0.000583784
      | 0.000394316
      | 0.000204847
      | 1.53782E-05
      | -0.000174091
      | -0.000363559
      | -0.000553028
      | 0.00056228
      | 0.000374724
      | 0.000187169
      | -3.86644E-07
      | -0.000187942
      | -0.000375498
      | -0.000563053
      | 0.000546298
      | 0.000362052
      | 0.000177806
      | -6.43933E-06
      | -0.000190685
      | -0.000374931
      | -0.000559176],[7,3])
  ZudX1 q+3 : Lookup_n-D  BreakpointsForDimension1=[-30 -20 -10 0 10 20 30]  BreakpointsForDimension2=[-35.0624 -15.3724 -13.8724]  BreakpointsForDimension3=[-5.14444 -3.08666664 -1.54332]  Table=|  InternalRulePriority=Speed  RndMeth=Simplest  InputSameDT=on
      | reshape([-0.000586989
      | -0.000395541
      | -0.000204094
      | -1.26467E-05
      | 0.000178801
      | 0.000370248
      | 0.000561695
      | -0.000568868
      | -0.000379268
      | -0.000189669
      | -6.86388E-08
      | 0.000189531
      | 0.000379131
      | 0.000568731
      | -0.000565299
      | -0.000378949
      | -0.000192598
      | -6.24776E-06
      | 0.000180103
      | 0.000366453
      | 0.000552804],[7,3])
  ZudX1 q+4 : Lookup_n-D  BreakpointsForDimension1=[-30 -20 -10 0 10 20 30]  BreakpointsForDimension2=[-35.0624 -15.3724 -13.8724]  BreakpointsForDimension3=[-5.14444 -3.08666664 -1.54332]  Table=|  InternalRulePriority=Speed  RndMeth=Simplest  InputSameDT=on
      | reshape([-0.000638396
      | -0.000426715
      | -0.000215035
      | -3.35454E-06
      | 0.000208326
      | 0.000420006
      | 0.000631687
      | -0.000598951
      | -0.000393944
      | -0.000188937
      | 1.60698E-05
      | 0.000221077
      | 0.000426084
      | 0.000631091
      | -0.000622514
      | -0.000421726
      | -0.000220939
      | -2.01522E-05
      | 0.000180635
      | 0.000381422
      | 0.000582209],[7,3])
  ZudX1 q+5 : Lookup_n-D  BreakpointsForDimension1=[-30 -20 -10 0 10 20 30]  BreakpointsForDimension2=[-35.0624 -15.3724 -13.8724]  BreakpointsForDimension3=[-35.0624 -15.3724 -13.8724]  Table=|  InternalRulePriority=Speed  RndMeth=Simplest  InputSameDT=on
      | reshape([-0.000461714
      | -0.000296336
      | -0.000130959
      | 3.44194E-05
      | 0.000199797
      | 0.000365175
      | 0.000530553
      | -0.000503641
      | -0.000327652
      | -0.000151663
      | 2.43257E-05
      | 0.000200315
      | 0.000376303
      | 0.000552292
      | -0.000536558
      | -0.000356664
      | -0.00017677
      | 3.1235E-06
      | 0.000183017
      | 0.000362911
      | 0.000542805],[7,3])
  MdX : Outport
  wires:
  Demux6/5 -> ZudX1 q+5/1
  Demux6/4 -> ZudX1 q+4/1
  Demux6/3 -> ZudX1 q+3/1
  Demux6/2 -> ZudX1 q+2/1
  ZudX1 q+4/1 -> Gain1/1
  ZudX1 q+3/1 -> Gain2/1
  ZudX1 q+2/1 -> Gain3/1
  ZudX1 q+1/1 -> Gain/1
  ZudX1 q+5/1 -> Gain4/1
  z/1 -> ZudX1 q+5/2, ZudX1 q+4/2, ZudX1 q+3/2, ZudX1 q+2/2, ZudX1 q+1/2
  Mux/1 -> MdX/1
  Demux6/1 -> ZudX1 q+1/1
  dX/1 -> Demux6/1
  Gain/1 -> Mux/1
  Gain3/1 -> Mux/2
  Gain2/1 -> Mux/3
  Gain1/1 -> Mux/4
  Gain4/1 -> Mux/5

== system Model_6DOF_B3_2019a/HDM/HDM B3/N/NdXi ==
  dX : Inport
  z : Inport  Port=2
  Mux : Mux
  NdX1 : Lookup_n-D  BreakpointsForDimension1=[-10 0 10]  BreakpointsForDimension2=|  BreakpointsForDimension3=[-5.14444 -3.08666664 -1.54332]  Table=|  InternalRulePriority=Speed  RndMeth=Simplest  InputSameDT=on
      BreakpointsForDimension2=|
      | [-36.4062987
      | -18.4062987
      | -15.4062987
      | -13.9062987]
      Table=|
      | reshape([-8.13475E-05
      | -3.25752E-06
      | 6.9363E-05
      | -8.00129E-05
      | -1.7093E-06
      | 7.14001E-05
      | -6.46417E-05
      | -1.7093E-06
      | 8.57128E-05
      | -7.85432E-05
      | -1.19372E-08
      | 7.37459E-05],[3,4])
  NdX2 : Lookup_n-D  BreakpointsForDimension1=[-10 0 10]  BreakpointsForDimension2=|  BreakpointsForDimension3=[-5.14444 -3.08666664 -1.54332]  Table=|  InternalRulePriority=Speed  RndMeth=Simplest  InputSameDT=on
      BreakpointsForDimension2=|
      | [-36.4062987
      | -18.4062987
      | -15.4062987
      | -13.9062987]
      Table=|
      | reshape([6.2278E-05
      | -3.5277E-06
      | -7.1028E-05
      | 5.9473E-05
      | -6.2352E-06
      | -7.5067E-05
      | 3.9525E-05
      | -6.2352E-06
      | -9.4282E-05
      | 5.5892E-05
      | -1.0640E-05
      | -8.2654E-05],[3,4])
  NdX3 : Lookup_n-D  BreakpointsForDimension1=[-10 0 10]  BreakpointsForDimension2=|  BreakpointsForDimension3=[-5.14444 -3.08666664 -1.54332]  Table=|  InternalRulePriority=Speed  RndMeth=Simplest  InputSameDT=on
      BreakpointsForDimension2=|
      | [-36.4062987
      | -18.4062987
      | -15.4062987
      | -13.9062987]
      Table=|
      | reshape([8.96891E-05
      | 3.65995E-06
      | -8.07998E-05
      | 9.13096E-05
      | 6.34009E-06
      | -7.59117E-05
      | 0.000100356
      | 6.34009E-06
      | -4.56822E-05
      | 9.40576E-05
      | 1.06795E-05
      | -6.79415E-05],[3,4])
  NdX4 : Lookup_n-D  BreakpointsForDimension1=[-10 0 10]  BreakpointsForDimension2=|  BreakpointsForDimension3=[-5.14444 -3.08666664 -1.54332]  Table=|  InternalRulePriority=Speed  RndMeth=Simplest  InputSameDT=on
      BreakpointsForDimension2=|
      | [-36.4062987
      | -18.4062987
      | -15.4062987
      | -13.9062987]
      Table=|
      | reshape([-7.16232E-05
      | 3.25314E-06
      | 8.32589E-05
      | -7.3213E-05
      | 1.68586E-06
      | 8.13825E-05
      | -8.66615E-05
      | 1.68586E-06
      | 6.54218E-05
      | -7.48528E-05
      | -6.7812E-08
      | 7.92559E-05],[3,4])
  Selector1 : Selector  InputPortWidth=5  IndexOptions=Index vector (dialog)  Indices=2  OutputSizes=1
  Selector2 : Selector  InputPortWidth=5  IndexOptions=Index vector (dialog)  Indices=3  OutputSizes=1
  Selector3 : Selector  InputPortWidth=5  IndexOptions=Index vector (dialog)  Indices=4  OutputSizes=1
  Selector7 : Selector  InputPortWidth=5  IndexOptions=Index vector (dialog)  Indices=1  OutputSizes=1
  NdXi : Outport
  wires:
  dX/1 -> Selector3/1, Selector2/1, Selector1/1, Selector7/1
  Selector7/1 -> NdX1/1
  Mux/1 -> NdXi/1
  z/1 -> NdX4/2, NdX3/2, NdX2/2, NdX1/2
  NdX1/1 -> Mux/1
  NdX2/1 -> Mux/2
  NdX3/1 -> Mux/3
  NdX4/1 -> Mux/4
  Selector1/1 -> NdX2/1
  Selector2/1 -> NdX3/1
  Selector3/1 -> NdX4/1

== system Model_6DOF_B3_2019a/HDM/HDM B3/Wave, Virtual Mass and Hydrostatic/Wave Particle Motions ==
  U_ship : Inport
  X_earth : Inport  Port=2
  CGi : Inport  Port=3
  CG : Inport  Port=4
  SeaState : Inport  Port=5
  dLCG : Inport  Port=6
  dX_CTRL : Inport  Port=7
  fwrite : Inport  Port=8
  Add : Sum  Inputs=+-
  Clock : Clock
  Constant : Constant  Value=3
  Constant1 : Constant  Value=Zb
  Constant2 : Constant  Value=0.474
  Constant6 : Constant  Value=1025
  Constant7 : Constant  Value=9.81
  Local eff. Depth : MATLAB Function  TreatAsAtomicUnit=on
  MATLAB Function1 : MATLAB Function  TreatAsAtomicUnit=on
  Mux : Mux  Inputs=5
  Sectional Position Vectors : MATLAB Function  TreatAsAtomicUnit=on
  Sectional Wave Particle & Rigid Body Velocities : MATLAB Function  TreatAsAtomicUnit=on
  Subsystem : Subsystem
  Wave Properties : MATLAB Function  TreatAsAtomicUnit=on
  Wave particle velocity at hull CG : MATLAB Function  TreatAsAtomicUnit=on
  X_SP1 : Constant  Value=[31.924; 3.861; -3.861;]
  X_SP2 : Constant  Value=[31.924; 3.861; 3.861;]
  X_SP3 : Constant  Value=[31.924; -3.861; 3.861;]
  X_SP4 : Constant  Value=[31.924; -3.861; -3.861;]
  X_XB : Constant  Value=[-10.465; 0; 9.732;]
  beta_wave : Constant  Value=0
  phi_wave : Constant  Value=0
  Rs : Outport
  zeff : Outport  Port=2
  uwXis : Outport  Port=3
  uwsCG : Outport  Port=4
  uws : Outport  Port=5
  urs : Outport  Port=6
  B_FM : Outport  Port=7
  wires:
  Sectional Position Vectors/2(Rs) -> Sectional Wave Particle & Rigid Body Velocities/5(Rs), Rs/1
  SeaState/1 -> Wave Properties/1(SeaState)
  Clock/1 -> MATLAB Function1/1(time), Wave particle velocity at hull CG/1(time), Local eff. Depth/1(time), Sectional Wave Particle & Rigid Body Velocities/1(time), Subsystem/1(time)
  Sectional Position Vectors/1(Xce) -> Sectional Wave Particle & Rigid Body Velocities/4(Xce)
  X_earth/1 -> Subsystem/2(Xearth), Sectional Wave Particle & Rigid Body Velocities/3(X_earth), MATLAB Function1/7(X_earth), Wave particle velocity at hull CG/2(X_earth), Local eff. Depth/2(Bxe), Sectional Position Vectors/1(X_earth)
  Wave Properties/3(k_wave) -> Subsystem/4(k_wave), Wave particle velocity at hull CG/8(k_wave), Local eff. Depth/3(k_wave), MATLAB Function1/13(k_wave), Sectional Wave Particle & Rigid Body Velocities/10(k_wave)  "k"
  U_ship/1 -> MATLAB Function1/8(U_ship), Sectional Wave Particle & Rigid Body Velocities/2(U_ship)
  Wave Properties/1(L_wave) -> MATLAB Function1/9(L_wave), Sectional Wave Particle & Rigid Body Velocities/8(L_wave), Wave particle velocity at hull CG/4(L_wave)
  Wave Properties/4(w_wave) -> Subsystem/5(w_wave), Wave particle velocity at hull CG/9(w_wave), Local eff. Depth/4(w_wave), MATLAB Function1/14(w_wave), Sectional Wave Particle & Rigid Body Velocities/11(w_wave)  "w"
  CGi/1 -> Sectional Position Vectors/2(CGi)
  CG/1 -> Sectional Position Vectors/3(CG)
  Sectional Wave Particle & Rigid Body Velocities/2(Urs) -> urs/1
  Sectional Wave Particle & Rigid Body Velocities/1(Uws) -> uws/1
  dLCG/1 -> Wave particle velocity at hull CG/3(dLCG), Sectional Position Vectors/4(dLCG)
  Wave Properties/2(A_wave) -> Subsystem/3(A_wave), Wave particle velocity at hull CG/7(A_wave), Local eff. Depth/5(a_wave), MATLAB Function1/12(A_wave), Sectional Wave Particle & Rigid Body Velocities/9(A_wave)
  Local eff. Depth/1(z_eff) -> zeff/1
  X_XB/1 -> MATLAB Function1/6(rXB)
  X_SP4/1 -> MATLAB Function1/5(rX4)
  X_SP3/1 -> MATLAB Function1/4(rX3)
  X_SP2/1 -> MATLAB Function1/3(rX2)
  X_SP1/1 -> MATLAB Function1/2(rX1)
  MATLAB Function1/1(uwX1s) -> Mux/1
  MATLAB Function1/2(uwX2s) -> Mux/2
  MATLAB Function1/3(uwX3s) -> Mux/3
  MATLAB Function1/4(uwX4s) -> Mux/4
  MATLAB Function1/5(uwXBs) -> Mux/5
  Mux/1 -> uwXis/1
  phi_wave/1 -> Sectional Wave Particle & Rigid Body Velocities/6(phi_wave), Wave particle velocity at hull CG/5(phi_wave), MATLAB Function1/10(phi_wave)
  beta_wave/1 -> MATLAB Function1/11(beta_wave), Sectional Wave Particle & Rigid Body Velocities/7(beta_wave), Wave particle velocity at hull CG/6(beta_wave)
  Wave particle velocity at hull CG/1(uwsCG) -> uwsCG/1
  Constant/1 -> Sectional Wave Particle & Rigid Body Velocities/12(iProbe)
  Subsystem/1(Out1) -> B_FM/1
  Constant6/1 -> Subsystem/6(rho)
  Constant7/1 -> Subsystem/7(g)
  Add/1 -> Subsystem/8(Zb)
  Constant2/1 -> Add/1
  Constant1/1 -> Add/2
  dX_CTRL/1 -> Subsystem/9(dX_CTRL)
  fwrite/1 -> Subsystem/10(fwrite)
